simulink model "TARCSimulation"  (R2025b)
settings: Solver=FixedStepAuto  StartTime=0.0  StopTime=5.2  FixedStep=0.001  RelTol=1e-3
model workspace (MAT data in the model file):
  RocketTotalWeight = 0.39973
undefined symbols (not defined in the file): ft, m, s
libraries: aerolibconvert2 x4
settings Model: PauseTimes=0.001  SnapshotBufferSize=100  SnapshotInterval=1  Creator=aditya  LastModifiedBy=aditya
settings HardwareCC: ProdBitPerLong=64.0  ProdHWDeviceType=Intel->x86-64 (Linux 64)

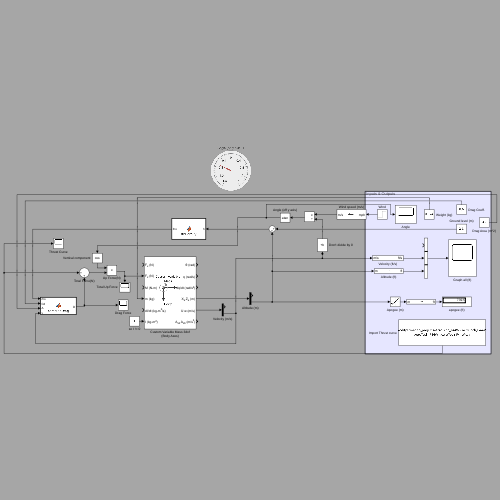
[thumbnail: Simulink's stored preview of the top-level diagram]
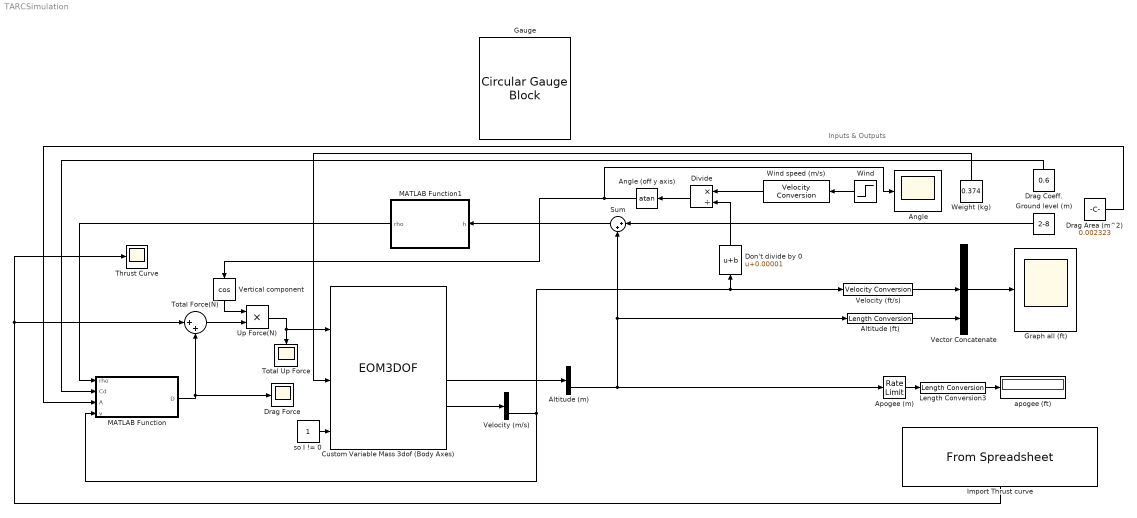
== system TARCSimulation ==
  note: Inputs & Outputs
  Altitude (ft) : aerolibconvert2/Length Conversion  IU=m  OU=ft
  Altitude (m) : Demux  Outputs=2
  Angle : Scope
      settings: ActiveDisplayYMinimum=-2.2460779532793387  ActiveDisplayYMaximum=2.6080118509564221
  Angle (off y axis) : Trigonometry  Operator=atan  ApproximationMethod=CORDIC
  Apogee (m) : RateLimiter  RisingSlewLimit=9999999999  FallingSlewLimit=0  SampleTimeMode=inherited
  Custom Variable Mass 3dof (Body Axes) : EOM3DOF  mtype=Custom Variable  v_ini=0  g=-9.81
  Divide : Product  Inputs=*/
  Don't divide by 0 : Bias  Bias=0.00001  SaturateOnIntegerOverflow=off
  Drag Area (m^2) : Constant  Value=0.002323
  Drag Coeff. : Constant  Value=0.6
  Drag Force : Scope
      settings: ActiveDisplayYMinimum=-1  ActiveDisplayYMaximum=1  DataLoggingVariableName=ScopeData2
  Gauge : CircularGaugeBlock  ScaleMin=-1.6  ScaleMax=1.6  FontColor=[0.0, 0.0, 0.0]
  Graph all (ft) : Scope
      settings: ActiveDisplayYMinimum=-182.13178650668624  ActiveDisplayYMaximum=999.03735352042611
  Ground level (m) : Constant  Value=2-8
  Import Thrust curve : FromSpreadsheet  FileName=/home/aditya/matlab_projects/AeroTech_F44W - AeroTech_F44W.csv.xls  SheetName=AeroTech_F44W - AeroTech_F44W.csv
  Length Conversion3 : aerolibconvert2/Length Conversion  IU=m  OU=ft
  MATLAB Function : MATLAB Function  TreatAsAtomicUnit=on
  MATLAB Function1 : MATLAB Function  TreatAsAtomicUnit=on
  Sum : Sum  Inputs=|++
  Thrust Curve : Scope
      settings: ActiveDisplayYMinimum=-1  ActiveDisplayYMaximum=1  DataLoggingVariableName=ScopeData4
  Total Force(N) : Sum  Inputs=|++
  Total Up Force : Scope
      settings: ActiveDisplayYMinimum=-36.236430858530035  ActiveDisplayYMaximum=72.28217553096647  DataLoggingVariableName=ScopeData3
  Up Force(N) : Product
  Vector Concatenate : Concatenate  NumInputs=3
  Velocity (ft/s) : aerolibconvert2/Velocity Conversion  IU=m/s  OU=ft/s
  Velocity (m/s) : Demux  Outputs=2
  Vertical component : Trigonometry  Operator=cos
  Weight (kg) : Constant  Value=0.374
  Wind : Step  Time=0.1  After=10  SampleTime=0
  Wind speed (m/s) : aerolibconvert2/Velocity Conversion  IU=mph  OU=m/s
  apogee (ft) : Display
  so I != 0 : Constant
  wires:
  Custom Variable Mass 3dof (Body Axes)/4 -> Altitude (m)/1
  Custom Variable Mass 3dof (Body Axes)/5 -> Velocity (m/s)/1
  MATLAB Function/1(D) -> Drag Force/1, Total Force(N)/2
  Weight (kg)/1 -> Custom Variable Mass 3dof (Body Axes)/4
  Import Thrust curve/1 -> Thrust Curve/1, Total Force(N)/1
  Ground level (m)/1 -> Sum/1
  Altitude (m)/2 -> Sum/2, Altitude (ft)/1, Apogee (m)/1
  Apogee (m)/1 -> Length Conversion3/1
  Altitude (ft)/1 -> Vector Concatenate/3
  Vector Concatenate/1 -> Graph all (ft)/1
  Velocity (ft/s)/1 -> Vector Concatenate/2
  Length Conversion3/1 -> apogee (ft)/1
  Drag Coeff./1 -> MATLAB Function/2(Cd)
  Sum/1 -> MATLAB Function1/1(h)
  MATLAB Function1/1(rho) -> MATLAB Function/1(rho)
  Wind/1 -> Wind speed (m/s)/1
  Vertical component/1 -> Up Force(N)/1
  Total Force(N)/1 -> Up Force(N)/2
  Up Force(N)/1 -> Custom Variable Mass 3dof (Body Axes)/2, Total Up Force/1
  so I != 0/1 -> Custom Variable Mass 3dof (Body Axes)/6
  Angle (off y axis)/1 -> Angle/1, Vertical component/1
  Divide/1 -> Angle (off y axis)/1
  Velocity (m/s)/2 -> MATLAB Function/4(v), Don't divide by 0/1, Velocity (ft/s)/1
  Wind speed (m/s)/1 -> Divide/1
  Don't divide by 0/1 -> Divide/2
  Drag Area (m^2)/1 -> MATLAB Function/3(A)

== matlab function TARCSimulation/MATLAB Function1 ==
  data: h input; rho output
function rho = airDensity(h)
% airDensity  Compute air density (kg/m^3) at a given altitude (m)
%
%   rho = airDensity(h)
%
%   Input:
%       h  - Altitude above mean sea level in meters (scalar or vector)
%
%   Output:
%       rho - Air density in kg/m^3
%
%   Model:
%       Based on the International Standard Atmosphere (ISA) up to 11 km.
%


    % --- Constants ---
    T0 = 288.15;      % Sea level standard temperature (K)
    p0 = 101325;      % Sea level standard pressure (Pa)
    L  = 0.0065;      % Temperature lapse rate (K/m)
    R  = 287.058;     % Specific gas constant for dry air (J/kg·K)
    g  = 9.80665;     % Gravitational acceleration (m/s^2)

    % --- Compute temperature at altitude ---
    T = T0 - L .* h;

    % Clamp for altitudes above tropopause (~11 km)
    T(T < 216.65) = 216.65;

    % --- Compute pressure using barometric formula ---
    p = p0 .* (T ./ T0) .^ (g / (R * L));

    % --- Compute density ---
    rho = p ./ (R .* T);

end

== matlab function TARCSimulation/MATLAB Function ==
  data: rho input; Cd input; A input; v input; D output
function D = computeDrag(rho, Cd, A, v)

D = -0.5 * Cd * rho * A * (v^2);
end
